simulink library "tqd"  (R2021b)
settings: Solver=VariableStepAuto  StartTime=0.0  StopTime=10.0  RelTol=1e-3
undefined symbols (not defined in the file or in its folder): ATQD_APSDecReq_X_kph, ATQD_APSDecReq_Y_mps2, ATQD_APSDecReqCMD_X_kph, ATQD_APSDecReqTs_X_pct, ATQD_APSDecTimeGain_X_Deg, ATQD_APSDecTimeGain_Y_s, ATQD_APSReqLowSpd_X_Deg, ATQD_AutoHoldReleaseBPS_X_Deg, ATQD_AWDLoadTrqnsGain_X_kg, ATQD_AWDLoadTrqnsGain_Y_pct, ATQD_BOSEnBPSPosn_X_kph, ATQD_BOSMap_X_rpm, ATQD_BOSMap_Y_pct, ATQD_CreepBaseTqD_X_kph, ATQD_CreepBaseTqD_Y_Deg, ATQD_CreepBaseTqR_X_kph, ATQD_CreepBaseTqR_Y_Deg, ATQD_CreepBPSDisPosn_X_Deg, ATQD_CreepBPSDisPosnR_X_Deg, ATQD_CreepBPSEnPosn_X_Deg, ATQD_CreepBPSEnPosnR_X_Deg, ATQD_CreepDeltaTq_X_kph, ATQD_CreepIterm_X_kph, ATQD_CreepIterm_Y_kph, ATQD_CreepItermMaxLimit_X_pct, ATQD_CreepPreloadTime_X_kph, ATQD_CreepPreloadTq_X_kph, ATQD_CreepPreloadTq_Y_s, ATQD_CreepProtTq_X_Deg, ATQD_CreepPterm_X_kph, ATQD_CreepPterm_Y_kph, ATQD_ECOTqMapD_X_rpm, ATQD_ECOTqMapD_Y_pct, ATQD_EOPDTqMapDCon_X_rpm, ATQD_EOPDTqMapDCon_Y_Deg, ATQD_EstInitVehWeight_X_c, ATQD_LHMRollGenMapD_X_rpm, ATQD_LHMRollGenMapD_Y_rpm, ATQD_LHMTqMapD_X_rpm, ATQD_LHMTqMapD_Y_pct, ATQD_NL1TqMapD_X_rpm, ATQD_NL1TqMapD_Y_pct, ATQD_NOPDTqMapDCon_X_rpm, ATQD_NOPDTqMapDCon_Y_Deg, ATQD_NRMRrEDUSpRat_X_rpm, ATQD_NRMRrEDUSpRat_Y_Nm, ATQD_OPDHoldDownRelDelay_X_Deg, ATQD_OPDHoldEnSpd_X_Deg, ATQD_OPDHoldRelDetTime_X_Deg, ATQD_OPDHoldReleaseTq_X_Deg, ATQD_OrigPedTqLowLim_X_Deg, ATQD_OrigPedTqLowLim_Y_pct, ATQD_PedalMapClimbUpLim_X_rpm, ATQD_PedalMapClimbUpLim_Y_Deg, ATQD_PreLoadTq_X_s, ATQD_RollGenMapEL1_X_rpm, ATQD_RollGenMapEL1_Y_rpm, ATQD_SL1TqMapD_X_rpm, ATQD_SL1TqMapD_Y_pct, ATQD_SlideRegenTqGain_X_Gps ... (+487)
libraries: hcu_lib x83, simulink x73, tqr x1
(part 10 of 19)

== system tqd/TQD/TorqueDemand/Signal_convert/VehWeightEst/Desicion ==
  task_time_s : Inport
  VTQD_VehWeightEstDis_flg : Inport  Port=2
  VTQD_EstVehWeight_kg : Inport  Port=3
  VINP_DriverSeatBeltCmd_flg : Inport  Port=4
  VINP_PsngrSeatBeltCmd_flg : Inport  Port=5
  VINP_RDriverSeatBeltCmd_flg : Inport  Port=6
  VINP_RCenterSeatBeltCmd_flg : Inport  Port=7
  VINP_RPsngrSeatBeltCmd_flg : Inport  Port=8
  VTQD_EstLongAccCheckPass_flg : Inport  Port=9
  VTQD_EstFrRealTqCheckPass_flg : Inport  Port=10
  VTQD_EstRrRealTqCheckPass_flg : Inport  Port=11
  AND : Logic  Inputs=5  AllPortsSameDT=off  OutDataTypeStr=boolean
  Add : Sum  Inputs=+++++
  Constant1 : Constant  Value=eps
  Constant{2,4,6,8,10} (5 alike) : Constant  Value=ZERO_INT
  Constant{3,5,7,9,11} (5 alike) : Constant  Value=ONE_INT
  Constant12 : Constant  Value=KTQD_EstEndDelayTime_s
  Data Type Conversion : DataTypeConversion  OutDataTypeStr=single
  Delay : Delay  DelayLength=1
  Delay1 : Delay  DelayLength=1
  DelayEnable : hcu_lib/Basic_Blocks/DelayEnable
  Equal : RelationalOperator  OutDataTypeStr=boolean  RndMeth=Simplest
  MTQD_EstInitVehWeight_Y_kg : Lookup_n-D  NumberOfTableDimensions=1  BreakpointsForDimension1=ATQD_EstInitVehWeight_X_c  Table=MTQD_EstInitVehWeight_Y_kg  ExtrapMethod=Clip  InternalRulePriority=Speed  RndMeth=Simplest  InputSameDT=on
  NOT : Logic  Operator=NOT  AllPortsSameDT=off  OutDataTypeStr=boolean
  Switch{,1..6} (7 alike) : Switch  Criteria=u2 > Threshold
  VTQD_VehWeightEstEnd_flg : Outport
  VTQD_EstVehWeightResult_kg : Outport  Port=2
  wires:
  Constant7/1 -> Switch4/1
  Constant1/1 -> Equal/2
  Switch2/1 -> Add/1
  [VINP_DriverSeatBeltCmd_flg] -> Switch2/2
  [VINP_RCenterSeatBeltCmd_flg] -> Switch4/2
  Switch5/1 -> Add/4
  Equal/1 -> Switch1/2
  Constant10/1 -> Switch6/3
  [VTQD_VehWeightEstDis_flg] -> AND/1
  Switch6/1 -> Add/5
  Delay/1 -> NOT/1
  Switch3/1 -> Add/2
  Constant6/1 -> Switch4/3
  Constant3/1 -> Switch2/1
  [VTQD_EstActVehWeight_kg] -> Switch1/1
  Constant2/1 -> Switch2/3
  [VTQD_VehWeightEstEnter_flg] -> Switch/2
  Constant11/1 -> Switch6/1
  Switch1/1 -> [VTQD_EstVehWeightResult_kg]  "VTQD_EstVehWeightResult_kg"
  Constant4/1 -> Switch3/3
  Constant5/1 -> Switch3/1
  [VINP_RDriverSeatBeltCmd_flg] -> Switch5/2
  Switch/1 -> Delay1/1, [VTQD_EstActVehWeight_kg]  "VTQD_EstActVehWeight_kg"
  AND/1 -> [VTQD_VehWeightEstEnter_flg]  "VTQD_VehWeightEstEnter_flg"
  [VINP_RPsngrSeatBeltCmd_flg] -> Switch6/2
  [VTQD_EstActVehWeight_kg] -> Equal/1
  [VINP_PsngrSeatBeltCmd_flg] -> Switch3/2
  Delay1/1 -> Switch/3
  [VTQD_EstInitVehWeight_kg] -> Switch1/3
  Constant9/1 -> Switch5/1
  Constant8/1 -> Switch5/3
  [VTQD_EstVehWeight_kg] -> Switch/1
  [VTQD_VehWeightEstEnd_flg] -> Delay/1
  NOT/1 -> AND/2
  Switch4/1 -> Add/3
  [VTQD_VehWeightEstDis_flg] -> DelayEnable/1
  Constant12/1 -> DelayEnable/2
  [task_time_s] -> DelayEnable/3
  DelayEnable/1 -> [VTQD_VehWeightEstEnd_flg]  "VTQD_VehWeightEstEnd_flg"
  task_time_s/1 -> [task_time_s]
  [VTQD_VehWeightEstEnd_flg] -> VTQD_VehWeightEstEnd_flg/1
  VTQD_VehWeightEstDis_flg/1 -> [VTQD_VehWeightEstDis_flg]
  VTQD_EstVehWeight_kg/1 -> [VTQD_EstVehWeight_kg]
  [VTQD_EstVehWeightResult_kg] -> VTQD_EstVehWeightResult_kg/1
  VINP_DriverSeatBeltCmd_flg/1 -> [VINP_DriverSeatBeltCmd_flg]
  VINP_PsngrSeatBeltCmd_flg/1 -> [VINP_PsngrSeatBeltCmd_flg]
  VINP_RDriverSeatBeltCmd_flg/1 -> [VINP_RDriverSeatBeltCmd_flg]
  VINP_RCenterSeatBeltCmd_flg/1 -> [VINP_RCenterSeatBeltCmd_flg]
  VINP_RPsngrSeatBeltCmd_flg/1 -> [VINP_RPsngrSeatBeltCmd_flg]
  VTQD_EstRrRealTqCheckPass_flg/1 -> [VTQD_EstRrRealTqCheckPass_flg]
  VTQD_EstFrRealTqCheckPass_flg/1 -> [VTQD_EstFrRealTqCheckPass_flg]
  VTQD_EstLongAccCheckPass_flg/1 -> [VTQD_EstLongAccCheckPass_flg]
  [VTQD_EstLongAccCheckPass_flg] -> AND/3
  [VTQD_EstFrRealTqCheckPass_flg] -> AND/4
  [VTQD_EstRrRealTqCheckPass_flg] -> AND/5
  MTQD_EstInitVehWeight_Y_kg/1 -> [VTQD_EstInitVehWeight_kg]  "VTQD_EstInitVehWeight_kg"
  Data Type Conversion/1 -> MTQD_EstInitVehWeight_Y_kg/1
  Add/1 -> Data Type Conversion/1  "VTQD_EstInitVehWightX_c"

== system tqd/TQD/TorqueDemand/TorqueModule/AvaliableTqLimit/If Action Subsystem1 ==
  VTQD_WhlTqCapGenF_Nm : Inport
  VTQD_WhlTqCapGenR_Nm : Inport  Port=2
  VTQD_DriverWhlTqDemFr_Nm : Inport  Port=3
  VTQD_DriverWhlTqDemRr_Nm : Inport  Port=4
  VVMC_ADASActive_flg : Inport  Port=5
  Action Port : ActionPort
  Constant{,1..3} (4 alike) : Constant  Value=ZERO_FLOAT
  Data Type Conversion1 : DataTypeConversion  OutDataTypeStr=single
  Data Type Conversion5 : DataTypeConversion  OutDataTypeStr=single
  Display : Display
  Display1 : Display
  Subtract : Sum  Inputs=+-
  Subtract1 : Sum  Inputs=+-
  Switch : Switch  Criteria=u2 > Threshold
  Switch1 : Switch  Criteria=u2 > Threshold
  Switch2 : Switch  Criteria=u2 ~= 0
  Switch3 : Switch  Criteria=u2 ~= 0
  VTQD_AvailTqWithARgnFr_Nm : Outport
  VTQD_AvailTqWithARgnRr_Nm : Outport  Port=2
  wires:
  Constant1/1 -> Switch1/1
  Constant/1 -> Switch/1
  Subtract1/1 -> Switch1/2, Switch1/3
  Subtract/1 -> Switch/2, Switch/3
  Switch1/1 -> Data Type Conversion5/1, VTQD_AvailTqWithARgnRr_Nm/1
  Switch/1 -> Data Type Conversion1/1, VTQD_AvailTqWithARgnFr_Nm/1
  VTQD_WhlTqCapGenR_Nm/1 -> Subtract1/1
  VTQD_WhlTqCapGenF_Nm/1 -> Subtract/1
  VTQD_DriverWhlTqDemFr_Nm/1 -> Switch2/3
  Switch2/1 -> Subtract/2
  Constant2/1 -> Switch2/1
  VVMC_ADASActive_flg/1 -> Switch3/2, Switch2/2
  Constant3/1 -> Switch3/1
  VTQD_DriverWhlTqDemRr_Nm/1 -> Switch3/3
  Switch3/1 -> Subtract1/2
  Data Type Conversion1/1 -> Display/1  "VTQD_AvailTqWithARgnFr_Nm"
  Data Type Conversion5/1 -> Display1/1  "VTQD_AvailTqWithARgnRr_Nm"

== system tqd/TQD/TorqueDemand/TorqueModule/AvaliableTqLimit/If Action Subsystem2 ==
  VTQD_WhlTqCapGenF_Nm : Inport
  VTQD_WhlTqCapGenR_Nm : Inport  Port=2
  Action Port : ActionPort
  Data Type Conversion4 : DataTypeConversion  OutDataTypeStr=single
  Data Type Conversion5 : DataTypeConversion  OutDataTypeStr=single
  Display : Display
  Display1 : Display
  VTQD_AvailTqNoARgnFr_Nm : Outport
  VTQD_AvailTqNoARgnRr_Nm : Outport  Port=2
  wires:
  VTQD_WhlTqCapGenF_Nm/1 -> Data Type Conversion4/1, VTQD_AvailTqNoARgnFr_Nm/1
  VTQD_WhlTqCapGenR_Nm/1 -> Data Type Conversion5/1, VTQD_AvailTqNoARgnRr_Nm/1
  Data Type Conversion4/1 -> Display/1  "VTQD_AvailTqNoARgnFr_Nm"
  Data Type Conversion5/1 -> Display1/1  "VTQD_AvailTqNoARgnRr_Nm"

== system tqd/TQD/TorqueDemand/TorqueModule/AvaliableTqLimit/TorqueCapacityCalcalation ==
  VTQD_FrShaftSpd_rpm : Inport
  VTQD_RrShaftSpd_rpm : Inport  Port=2
  VINP_HVBPwrAvailDchrg_kw : Inport  Port=3
  VINP_HVBPwrAvailChrg_kw : Inport  Port=4
  KTQD_FrBatapCont_factor : Inport  Port=5
  KTQD_RrBatapCont_factor : Inport  Port=6
  VTQD_FrEDUSpRat_cmd : Inport  Port=7
  VTQD_RrEDUSpRat_rat : Inport  Port=8
  VINP_FrMotorAvailTq_Nm : Inport  Port=9
  VINP_RrMotorAvailTq_Nm : Inport  Port=10
  VINP_HVBCellVoltMax_mV : Inport  Port=11
  VINP_HVBCellVoltMin_mV : Inport  Port=12
  VINP_HVBSOH_pct : Inport  Port=13
  VINP_FrRegenAvailTq_Nm : Inport  Port=14
  VINP_RrRegenAvailTq_Nm : Inport  Port=15
  VTQD_GearActualPosn_enum : Inport  Port=16
  VINP_VehicleType_enum : Inport  Port=17
  CapacityDistribution : Subsystem
  Generation : Subsystem
  Motoring : Subsystem
  TMAvailablePwr_Calculation : Subsystem
  VTQD_WhlTqCapMotFr_Nm : Outport
  VTQD_WhlTqCapMotRr_Nm : Outport  Port=2
  VTQD_WhlTqCapGenFr_Nm : Outport  Port=3
  VTQD_WhlTqCapGenRr_Nm : Outport  Port=4
  wires:
  [VTQD_TMPwrAvailDchrg_kW] -> CapacityDistribution/3(VTQD_TMPwrAvailDchrg_kW)
  TMAvailablePwr_Calculation/1(VTQD_TMPwrAvailDchrg_kW) -> [VTQD_TMPwrAvailDchrg_kW]
  [VINP_HVBPwrAvailDchrg_kw] -> TMAvailablePwr_Calculation/1(VINP_HVBPwrAvailDchrg_kw)
  Motoring/2(VTQD_WhlTqCapMotRr_Nm) -> VTQD_WhlTqCapMotRr_Nm/1
  [VTQD_RrEDUSpRat_rat] -> CapacityDistribution/2(VTQD_RrEDUSpRat_rat)
  [VTQD_FrEDUSpRat_rat] -> CapacityDistribution/1(VTQD_FrEDUSpRat_cmd)
  CapacityDistribution/4(VTQD_RrHVBPwrAvailChrg_kw) -> [VTQD_RrHVBPwrAvailChrg_kw]
  CapacityDistribution/3(VTQD_FrHVBPwrAvailChrg_kw) -> [VTQD_FrHVBPwrAvailChrg_kw]
  CapacityDistribution/2(VTQD_RrHVBPwrAvailDchrg_kw) -> [VTQD_RrHVBPwrAvailDchrg_kw]
  CapacityDistribution/1(VTQD_FrHVBPwrAvailDchrg_kw) -> [VTQD_FrHVBPwrAvailDchrg_kw]
  [VINP_HVBPwrAvailChrg_kw] -> CapacityDistribution/4(VINP_HVBPwrAvailChrg_kw)
  [VTQD_RrHVBPwrAvailChrg_kw] -> Generation/4(VTQD_RrHVBPwrAvailChrg_kw)
  [KTQD_RrBatapCont_factor] -> Generation/6(KTQD_RrBatapCont_factor)
  [VTQD_FrShaftSpd_rpm] -> Generation/1(VTQD_FrShaftSpd_rpm)
  [VTQD_FrHVBPwrAvailChrg_kw] -> Generation/3(VTQD_FrHVBPwrAvailChrg_kw)
  [VTQD_RrShaftSpd_rpm] -> Generation/2(VTQD_RrShaftSpd_rpm)
  [KTQD_FrBatapCont_factor] -> Generation/5(KTQD_FrBatapCont_factor)
  Generation/1(VTQD_WhlTqCapGenFr_Nm) -> VTQD_WhlTqCapGenFr_Nm/1
  Generation/2(VTQD_WhlTqCapGenRr_Nm) -> VTQD_WhlTqCapGenRr_Nm/1
  [VTQD_RrHVBPwrAvailDchrg_kw] -> Motoring/4(VTQD_RrHVBPwrAvailDchrg_kw)
  [VTQD_FrHVBPwrAvailDchrg_kw] -> Motoring/3(VTQD_FrHVBPwrAvailDchrg_kw)
  [KTQD_RrBatapCont_factor] -> Motoring/6(KTQD_RrBatapCont_factor)
  VTQD_RrEDUSpRat_rat/1 -> [VTQD_RrEDUSpRat_rat]
  VTQD_FrEDUSpRat_cmd/1 -> [VTQD_FrEDUSpRat_rat]
  KTQD_RrBatapCont_factor/1 -> [KTQD_RrBatapCont_factor]
  [VTQD_RrShaftSpd_rpm] -> Motoring/2(VTQD_RrShaftSpd_rpm)
  VTQD_RrShaftSpd_rpm/1 -> [VTQD_RrShaftSpd_rpm]
  VTQD_FrShaftSpd_rpm/1 -> [VTQD_FrShaftSpd_rpm]
  VINP_HVBPwrAvailChrg_kw/1 -> [VINP_HVBPwrAvailChrg_kw]
  VINP_HVBPwrAvailDchrg_kw/1 -> [VINP_HVBPwrAvailDchrg_kw]
  KTQD_FrBatapCont_factor/1 -> [KTQD_FrBatapCont_factor]
  [VTQD_FrShaftSpd_rpm] -> Motoring/1(VTQD_FrShaftSpd_rpm)
  Motoring/1(VTQD_WhlTqCapMotFr_Nm) -> VTQD_WhlTqCapMotFr_Nm/1
  [KTQD_FrBatapCont_factor] -> Motoring/5(KTQD_FrBatapCont_factor)
  VINP_HVBSOH_pct/1 -> [VINP_HVBSOH_pct]
  VINP_HVBCellVoltMin_mV/1 -> [VINP_HVBCellVoltMin_mV]
  VINP_HVBCellVoltMax_mV/1 -> [VINP_HVBCellVoltMax_mV]
  [VINP_HVBSOH_pct] -> Motoring/9(VINP_HVBSOH_pct)
  [VINP_HVBCellVoltMin_mV] -> Motoring/8(VINP_HVBCellVoltMin_mV)
  [VINP_HVBCellVoltMax_mV] -> Motoring/7(VINP_HVBCellVoltMax_mV)
  [VINP_RrMotorAvailTq_Nm] -> Motoring/11(VINP_RrMotorAvailTq_Nm)
  [VINP_FrMotorAvailTq_Nm] -> Motoring/10(VINP_FrMotorAvailTq_Nm)
  [VINP_FrRegenAvailTq_Nm] -> Generation/7(VINP_FrRegenAvailTq_Nm)
  [VINP_RrRegenAvailTq_Nm] -> Generation/8(VINP_RrRegenAvailTq_Nm)
  VINP_RrRegenAvailTq_Nm/1 -> [VINP_RrRegenAvailTq_Nm]
  VINP_FrRegenAvailTq_Nm/1 -> [VINP_FrRegenAvailTq_Nm]
  VINP_FrMotorAvailTq_Nm/1 -> [VINP_FrMotorAvailTq_Nm]
  VINP_RrMotorAvailTq_Nm/1 -> [VINP_RrMotorAvailTq_Nm]
  [VTQD_GearActualPosn_enum] -> Motoring/12(VTQD_GearActualPosn_enum)
  [VTQD_GearActualPosn_enum] -> Generation/9(VTQD_GearActualPosn_enum)
  VTQD_GearActualPosn_enum/1 -> [VTQD_GearActualPosn_enum]
  [VINP_VehicleType_enum] -> Motoring/13(VINP_VehicleType_enum)
  [VINP_VehicleType_enum] -> Generation/10(VINP_VehicleType_enum)
  VINP_VehicleType_enum/1 -> [VINP_VehicleType_enum]

== system tqd/TQD/TorqueDemand/TorqueModule/DriverWhlTqDem/BOS ==
  VTQD_ActBPSPosn_pct : Inport
  VTQD_TqTargetShaftSpd_rpm : Inport  Port=2
  VTQD_VehActSpd_kph : Inport  Port=3
  VTQD_PedalMapWhlTq_Nm : Inport  Port=4
  VTQD_CreepBaseTqR_Nm : Inport  Port=5
  VTQD_CreepBaseTqD_Nm : Inport  Port=6
  VTQD_GearActualPosn_enum : Inport  Port=7
  VVMC_APSActive_flg : Inport  Port=8
  VTQD_LowIdleAccPedal_flg : Inport  Port=9
  VTQD_HighBPSPosn_flg : Inport  Port=10
  VTQD_BrkSwSta_flg : Inport  Port=11
  AND : Logic  Inputs=4  AllPortsSameDT=off  OutDataTypeStr=boolean
  AND1 : Logic  AllPortsSameDT=off  OutDataTypeStr=boolean
  AND2 : Logic  AllPortsSameDT=off  OutDataTypeStr=boolean
  Constant1 : Constant  Value=KTQD_BOSEnPedalTq_Nm
  Constant18 : Constant  Value=ZERO_FLOAT
  Constant20 : Constant  Value=ENUM_GEARACTUALPOSN_R
  Constant3 : Constant  Value=ONE_PERCENT
  Detect Change : simulink/Logic and Bit Operations/Detect Change  vinit=0  OutDataTypeStr=boolean
  Equal10 : RelationalOperator  Operator===  OutDataTypeStr=boolean  RndMeth=Simplest
  MTQD_BOSEnBPSPosn_Y_pct : Lookup_n-D  NumberOfTableDimensions=1  BreakpointsForDimension1=ATQD_BOSEnBPSPosn_X_kph  Table=MTQD_BOSEnBPSPosn_Y_pct  InternalRulePriority=Speed  RndMeth=Simplest  InputSameDT=on
  MTQD_BOSMap_Z_pct : Lookup_n-D  BreakpointsForDimension1=ATQD_BOSMap_Y_pct  BreakpointsForDimension2=ATQD_BOSMap_X_rpm  Table=MTQD_BOSMap_Z_pct  ExtrapMethod=Clip  InternalRulePriority=Speed  RndMeth=Simplest  InputSameDT=on
      settings: InputPortMap=u0,u1
  Max : MinMax  Function=max  Inputs=2
  NOT{,1..3} (4 alike) : Logic  Operator=NOT  AllPortsSameDT=off  OutDataTypeStr=boolean
  OR : Logic  Operator=OR  Inputs=3  AllPortsSameDT=off  OutDataTypeStr=boolean
  OR1 : Logic  Operator=OR  AllPortsSameDT=off  OutDataTypeStr=boolean
  Product1 : Product  RndMeth=Zero
  Product2 : Product  RndMeth=Zero
  Product3 : Product  RndMeth=Zero
  Relational Operator : RelationalOperator  Operator=>  OutDataTypeStr=boolean  RndMeth=Simplest
  Relational Operator1 : RelationalOperator  Operator=>  OutDataTypeStr=boolean  RndMeth=Simplest
  Relational Operator2 : RelationalOperator  OutDataTypeStr=boolean  RndMeth=Simplest
  Relational Operator5 : RelationalOperator  Operator=>  OutDataTypeStr=boolean  RndMeth=Simplest
  SR_Latch : hcu_lib/Basic_Blocks/SR_Latch
  Switch7 : Switch  Criteria=u2 > Threshold
  Switch8 : Switch  Criteria=u2 > Threshold
  VTQD_BOSEnable_flg : Outport
  VTQD_BOSTq_Nm : Outport  Port=2
  wires:
  VTQD_TqTargetShaftSpd_rpm/1 -> [VTQD_TqTargetShaftSpd_rpm]
  [VTQD_ActBPSPosn_pct] -> MTQD_BOSMap_Z_pct/1
  [VTQD_TqTargetShaftSpd_rpm] -> MTQD_BOSMap_Z_pct/2
  Constant3/1 -> Product1/2
  Product1/1 -> [VTQD_BOSReduction_gain]  "VTQD_BOSReduction_gain"
  MTQD_BOSMap_Z_pct/1 -> Product1/1
  VTQD_ActBPSPosn_pct/1 -> [VTQD_ActBPSPosn_pct]
  Relational Operator/1 -> AND/1
  VTQD_VehActSpd_kph/1 -> [VTQD_VehActSpd_kph]
  [VTQD_VehActSpd_kph] -> MTQD_BOSEnBPSPosn_Y_pct/1
  MTQD_BOSEnBPSPosn_Y_pct/1 -> Relational Operator/2  "VTQD_BOSEnBPSPosn_pct"
  [VTQD_ActBPSPosn_pct] -> Relational Operator/1
  VTQD_PedalMapWhlTq_Nm/1 -> [VTQD_PedalMapWhlTq_Nm]
  Relational Operator1/1 -> AND/2
  [VTQD_PedalMapWhlTq_Nm] -> Relational Operator1/1
  Constant1/1 -> Relational Operator1/2
  [VTQD_PedalMapWhlTq_Nm] -> Product2/1
  [VTQD_BOSReduction_gain] -> Product2/2
  Product3/1 -> Max/2
  Switch8/1 -> VTQD_BOSTq_Nm/1, [VTQD_BOSTq_Nm]  "VTQD_BOSTq_Nm"
  [VTQD_CreepBaseTqR_Nm] -> Switch7/1
  Max/1 -> Switch8/1
  Product2/1 -> Switch8/3
  Equal10/1 -> Switch7/2
  [VTQD_PedalMapWhlTq_Nm] -> Product3/1
  [VTQD_BOSReduction_gain] -> Product3/2
  [VTQD_GearActualPosn_enum] -> Equal10/1
  Relational Operator5/1 -> Switch8/2
  Constant20/1 -> Equal10/2
  Switch7/1 -> Max/1
  Constant18/1 -> Relational Operator5/2
  [VTQD_CreepBaseTqD_Nm] -> Switch7/3
  VTQD_CreepBaseTqD_Nm/1 -> [VTQD_CreepBaseTqD_Nm]
  VTQD_CreepBaseTqR_Nm/1 -> [VTQD_CreepBaseTqR_Nm]
  VTQD_GearActualPosn_enum/1 -> [VTQD_GearActualPosn_enum]
  [VTQD_BOSReduction_gain] -> Relational Operator5/1
  NOT/1 -> AND/3
  [VVMC_APSActive_flg] -> NOT/1
  VVMC_APSActive_flg/1 -> [VVMC_APSActive_flg]
  VTQD_LowIdleAccPedal_flg/1 -> [VTQD_LowIdleAccPedal_flg]
  [VTQD_LowIdleAccPedal_flg] -> NOT2/1
  NOT2/1 -> AND/4
  [VTQD_BrkSwSta_flg] -> NOT3/1
  AND2/1 -> OR/3
  AND1/1 -> OR1/1
  Detect Change/1 -> OR1/2
  Relational Operator2/1 -> OR/1
  [VTQD_LowIdleAccPedal_flg] -> AND2/1
  [VTQD_GearActualPosn_enum] -> Detect Change/1
  OR1/1 -> SR_Latch/2
  NOT3/1 -> AND2/2
  SR_Latch/1 -> VTQD_BOSEnable_flg/1  "VTQD_BOSEnable_flg"
  AND/1 -> NOT1/1, SR_Latch/1
  [VTQD_HighBPSPosn_flg] -> OR/2
  OR/1 -> AND1/2
  NOT1/1 -> AND1/1
  [VTQD_PedalMapWhlTq_Nm] -> Relational Operator2/1
  [VTQD_BOSTq_Nm] -> Relational Operator2/2
  VTQD_BrkSwSta_flg/1 -> [VTQD_BrkSwSta_flg]
  VTQD_HighBPSPosn_flg/1 -> [VTQD_HighBPSPosn_flg]

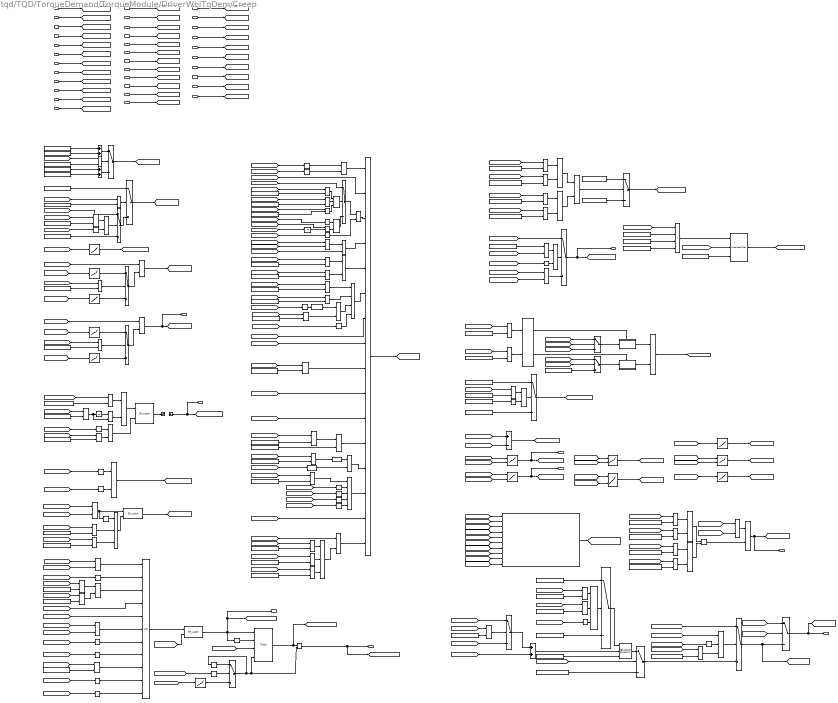
== system tqd/TQD/TorqueDemand/TorqueModule/DriverWhlTqDem/Creep ==
  note: Creep Enable Judgement
  note: Vehicle Actual Speed Calculation
  note: Creep Wheel Torque Demand Calculation
  VTQD_CreepON_flg : Inport
  VTQD_GearActualPosn_enum : Inport  Port=2
  VTQD_LowIdleAccPedal_flg : Inport  Port=3
  VINP_VehSpeed_kph : Inport  Port=4
  VTQD_TMRotateDirction_enum : Inport  Port=5
  VTQD_RegenMode_enum : Inport  Port=6
  VTQD_ActBPSPosn_pct : Inport  Port=7
  VTQD_PedalMapWhlTq_Nm : Inport  Port=8
  VINP_RrRBCActive_flg : Inport  Port=9
  VINP_FrRBCActive_flg : Inport  Port=10
  VVMC_ADASActive_flg : Inport  Port=11
  task_time_s : Inport  Port=12
  VTQD_LoSpdBrkCtrl_flg : Inport  Port=13
  VINP_AVHActive_flg : Inport  Port=14
  VTQD_APSReq_enum : Inport  Port=15
  VVMC_APSSpeedCMD_kph : Inport  Port=16
  VVMC_APSActive_flg : Inport  Port=17
  VTQD_RDCActive_enum : Inport  Port=18
  VVMC_APSReq_enum : Inport  Port=19
  " VINP_FrEDURealTMTq_Nm" : Inport  Port=20
  VINP_RrEDURealTMTq_Nm : Inport  Port=21
  VTQD_PreLoadPreEn_flg : Inport  Port=22
  VVMC_EstSlope_Deg : Inport  Port=23
  VPMM_PwrSta_enum : Inport  Port=24
  VTQD_TqTargetShaftSpd_rpm : Inport  Port=25
  VTQD_APSReqTimer_s : Inport  Port=26
  VINP_EPBSta_enum : Inport  Port=27
  VTQD_OPDHoldEnRel_flg : Inport  Port=28
  VTQD_ActAPSPosn_pct : Inport  Port=29
  VVMC_CAASActive_flg : Inport  Port=30
  VDDM_EPB1NoComCFS_flg : Inport  Port=31
  VDDM_EPB1RCErrCFS_flg : Inport  Port=32
  VDDM_EPB1CSErrCFS_flg : Inport  Port=33
  VDDM_EPBSigErrCFS_flg : Inport  Port=34
  AND{,1..2,4..7,9,11..12,15..16} (12 alike) : Logic  AllPortsSameDT=off  OutDataTypeStr=boolean
  AND10 : Logic  Operator=OR  AllPortsSameDT=off  OutDataTypeStr=boolean
  AND{3,8,13..14} (4 alike) : Logic  Inputs=3  AllPortsSameDT=off  OutDataTypeStr=boolean
  Add : Sum  Inputs=+-
  Add1 : Sum
  Add2 : Sum
  Add4 : Sum
  Constant1 : Constant  Value=KTQD_APSCMDEnCreepSpd_kph
  Constant10 : Constant  Value=KTQD_CreepTargetSpdR_kph
  Constant{3,11..12,21,25,58,62} (7 alike) : Constant  Value=ENUM_GEARACTUALPOSN_D
  Constant13 : Constant  Value=KTQD_CreepEnableSpd_kph
  Constant14 : Constant  Value=RPM2RADPS
  Constant15 : Constant  Value=ZERO_FLOAT
  Constant16 : Constant  Value=KTQD_TireRadius_m
  Constant17 : Constant  Value=ENUM_RDCACTSTA_NOREQUEST
  Constant18 : Constant  Value=ENUM_APSREQ_DECELCTRL  OutDataTypeStr=uint8
  Constant19 : Constant  Value=MPS2KPH
  Constant{2,9,20,31,35..36,38,42..44} (10 alike) : Constant  Value=ENUM_GEARACTUALPOSN_R
  Constant22 : Constant  Value=KTQD_CreepLowLimitTq_Nm
  Constant23 : Constant  Value=KTQD_CreepPrLoadEnSpd_kph
  Constant24 : Constant  Value=ENUM_RDCACTSTA_NOREQUEST
  Constant26 : Constant  Value=KTQD_CreepDisableSpdofst_kph
  Constant27 : Constant  Value=KTQD_CreepEnableSpdR_kph
  Constant28 : Constant  Value=KTQD_CreepDisableSpdofstR_kph
  Constant29 : Constant  Value=KTQD_CreepEnableSpdR_kph
  Constant30 : Constant  Value=ENUM_TMROTATEDIRECTACT_REVERSE  OutDataTypeStr=Inherit: Inherit via back propagation
  Constant32 : Constant  Value=ENUM_TMROTATEDIRECTACT_FORWARD  OutDataTypeStr=Inherit: Inherit via back propagation
  Constant33 : Constant  Value=KTQD_VehActSpdNegGain_gain
  Constant34 : Constant  Value=KTQD_VehActSpdPosGain_gain
  Constant37 : Constant  Value=ENUM_TMROTATEDIRECTACT_REVERSE  OutDataTypeStr=Inherit: Inherit via back propagation
  Constant39 : Constant  Value=ENUM_TMROTATEDIRECTACT_FORWARD  OutDataTypeStr=Inherit: Inherit via back propagation
  Constant{4,8,52,54,59,64} (6 alike) : Constant  Value=ENUM_REGENLEVEL_OPD
  Constant40 : Constant  Value=KTQD_RBCCreepRecTq_Nm
  Constant41 : Constant  Value=KTQD_RBCCreepRecTq_Nm
  Constant45 : Constant  Value=ENUM_POWERSTA_READY
  Constant46 : Constant  Value=KTQD_CreepEnableSpd_kph
  Constant47 : Constant  Value=KTQD_RPM2VehSpdTs_c
  Constant48 : Constant  Value=KTQD_CreepVehSpdSW_flg
  Constant49 : Constant  Value=KTQD_CreepTargetSpdD_kph
  Constant5 : Constant  Value=ENUM_APSREQ_BRKHOLD  OutDataTypeStr=uint8
  Constant50 : Constant  Value=KTQD_OPDCreepTargetSpdD_kph
  Constant51 : Constant  Value=KTQD_APSReqDisCreep_flg  OutDataTypeStr=uint8
  Constant53 : Constant  Value=KTQD_APSReqDelayTime_s
  Constant55 : Constant  Value=ENUM_EPBSTA_APPLIED  OutDataTypeStr=uint8
  Constant56 : Constant  Value=KTQD_APSReqDisCreep_flg
  Constant57 : Constant  Value=KTQD_CreepUpLimitTq_Nm
  Constant6 : Constant  Value=ENUM_GEARACTUALPOSN_P
  Constant60 : Constant  Value=KTQD_OPDCreepDUpLimitTq_Nm
  Constant61 : Constant  Value=KTQD_CreepDisPedTqSpd_kph
  Constant63 : Constant  Value=KTQD_CreepAPSPosn2Launch_pct
  Constant65 : Constant  Value=ENUM_APSREQ_DECELCTRL  OutDataTypeStr=uint8
  Constant7 : Constant  Value=ENUM_GEARACTUALPOSN_N
  Data Type Conversion : DataTypeConversion
  Delay : Delay  DelayLength=1
  Delay1 : Delay  DelayLength=1
  Detect Change : simulink/Logic and Bit Operations/Detect Change  vinit=0  OutDataTypeStr=boolean
  Detect Increase : simulink/Logic and Bit Operations/Detect Increase  vinit=0.0  OutDataTypeStr=boolean
  Equal{,1..4,6..8,10..16,19..31,33..39} (35 alike) : RelationalOperator  Operator===  OutDataTypeStr=boolean  RndMeth=Simplest
  Equal17 : RelationalOperator  Operator=<=  OutDataTypeStr=boolean  RndMeth=Simplest
  Equal18 : RelationalOperator  Operator=~=  OutDataTypeStr=boolean  RndMeth=Simplest
  Equal32 : RelationalOperator  OutDataTypeStr=boolean  RndMeth=Simplest
  Equal5 : RelationalOperator  Operator=<=  OutDataTypeStr=boolean  RndMeth=Simplest
  Equal9 : RelationalOperator  Operator=<=  OutDataTypeStr=boolean  RndMeth=Simplest
  FirstOrderFilter : hcu_lib/Basic_Blocks/FirstOrderFilter
  GreaterThan : RelationalOperator  Operator=>  OutDataTypeStr=boolean  RndMeth=Simplest
  GreaterThan1 : RelationalOperator  Operator=>  OutDataTypeStr=boolean  RndMeth=Simplest
  GreaterThan2 : RelationalOperator  OutDataTypeStr=boolean  RndMeth=Simplest
  GreaterThan3 : RelationalOperator  Operator=>  OutDataTypeStr=boolean  RndMeth=Simplest
  GreaterThan4 : RelationalOperator  Operator=<=  OutDataTypeStr=boolean  RndMeth=Simplest
  Ground2 : Ground
  If : If  NumInputs=2  IfExpression=u1 ~= 0  ElseIfExpressions=u2 ~= 0  ShowElse=off
  If Action Subsystem : Subsystem  TreatAsAtomicUnit=on
  If Action Subsystem1 : Subsystem  TreatAsAtomicUnit=on
  LiuzgSwitch1 : Switch  Criteria=u2 ~= 0
      settings: AttributesFormatString=<%<Criteria>>
  Logical Operator{,2,4,6} (4 alike) : Logic  AllPortsSameDT=off  OutDataTypeStr=boolean
  Logical Operator1 : Logic  Operator=OR  AllPortsSameDT=off  OutDataTypeStr=boolean
  Logical Operator{8..11} (4 alike) : Logic  Operator=NOT  AllPortsSameDT=off  OutDataTypeStr=boolean
  Logical Operator3 : Logic  Inputs=11  AllPortsSameDT=off  OutDataTypeStr=boolean
  Logical Operator5 : Logic  Operator=OR  AllPortsSameDT=off  OutDataTypeStr=boolean
  Logical Operator7 : Logic  Inputs=5  AllPortsSameDT=off  OutDataTypeStr=boolean
  MTQD_CreepBPSDisPosnR_Y_pct : Lookup_n-D  NumberOfTableDimensions=1  BreakpointsForDimension1=ATQD_CreepBPSDisPosnR_X_Deg  Table=MTQD_CreepBPSDisPosnR_Y_pct  ExtrapMethod=Clip  InternalRulePriority=Speed  RndMeth=Simplest  InputSameDT=on
  MTQD_CreepBPSDisPosn_Y_pct : Lookup_n-D  NumberOfTableDimensions=1  BreakpointsForDimension1=ATQD_CreepBPSDisPosn_X_Deg  Table=MTQD_CreepBPSDisPosn_Y_pct  ExtrapMethod=Clip  InternalRulePriority=Speed  RndMeth=Simplest  InputSameDT=on
  MTQD_CreepBPSEnPosnR_Y_pct : Lookup_n-D  NumberOfTableDimensions=1  BreakpointsForDimension1=ATQD_CreepBPSEnPosnR_X_Deg  Table=MTQD_CreepBPSEnPosnR_Y_pct  ExtrapMethod=Clip  InternalRulePriority=Speed  RndMeth=Simplest  InputSameDT=on
  MTQD_CreepBPSEnPosn_Y_pct : Lookup_n-D  NumberOfTableDimensions=1  BreakpointsForDimension1=ATQD_CreepBPSEnPosn_X_Deg  Table=MTQD_CreepBPSEnPosn_Y_pct  ExtrapMethod=Clip  InternalRulePriority=Speed  RndMeth=Simplest  InputSameDT=on
  MTQD_CreepBaseTqD_Z_Nm : Lookup_n-D  BreakpointsForDimension1=ATQD_CreepBaseTqD_Y_Deg  BreakpointsForDimension2=ATQD_CreepBaseTqD_X_kph  Table=MTQD_CreepBaseTqD_Z_Nm  ExtrapMethod=Clip  InternalRulePriority=Speed  RndMeth=Simplest  InputSameDT=on
      settings: InputPortMap=u0,u1
  MTQD_CreepBaseTqR_Z_Nm : Lookup_n-D  BreakpointsForDimension1=ATQD_CreepBaseTqR_Y_Deg  BreakpointsForDimension2=ATQD_CreepBaseTqR_X_kph  Table=MTQD_CreepBaseTqR_Z_Nm  ExtrapMethod=Clip  InternalRulePriority=Speed  RndMeth=Simplest  InputSameDT=on
      settings: InputPortMap=u0,u1
  MTQD_CreepDeltaTq_Y_Nm : Lookup_n-D  NumberOfTableDimensions=1  BreakpointsForDimension1=ATQD_CreepDeltaTq_X_kph  Table=MTQD_CreepDeltaTq_Y_Nm  ExtrapMethod=Clip  InternalRulePriority=Speed  RndMeth=Simplest  InputSameDT=on
  MTQD_CreepIterm_Z_Nm : Lookup_n-D  BreakpointsForDimension1=ATQD_CreepIterm_Y_kph  BreakpointsForDimension2=ATQD_CreepIterm_X_kph  Table=MTQD_CreepIterm_Z_Nm  ExtrapMethod=Clip  InternalRulePriority=Speed  RndMeth=Simplest  InputSameDT=on
      settings: InputPortMap=u0,u1
  MTQD_CreepPrelaodTq_Z_Nm : Lookup_n-D  BreakpointsForDimension1=ATQD_CreepPreloadTq_Y_s  BreakpointsForDimension2=ATQD_CreepPreloadTq_X_kph  Table=MTQD_CreepPreloadTq_Z_Nm  ExtrapMethod=Clip  InternalRulePriority=Speed  RndMeth=Simplest  InputSameDT=on
      settings: InputPortMap=u0,u1
  MTQD_CreepPreloadTime_Y_s : Lookup_n-D  NumberOfTableDimensions=1  BreakpointsForDimension1=ATQD_CreepPreloadTime_X_kph  Table=MTQD_CreepPreloadTime_Y_s  ExtrapMethod=Clip  InternalRulePriority=Speed  RndMeth=Simplest  InputSameDT=on
  MTQD_CreepProtTq_Y_Nm : Lookup_n-D  NumberOfTableDimensions=1  BreakpointsForDimension1=ATQD_CreepProtTq_X_Deg  Table=MTQD_CreepProtTq_Y_Nm  ExtrapMethod=Clip  InternalRulePriority=Speed  RndMeth=Simplest  InputSameDT=on
  MTQD_CreepPterm_Z_Nm : Lookup_n-D  BreakpointsForDimension1=ATQD_CreepPterm_Y_kph  BreakpointsForDimension2=ATQD_CreepPterm_X_kph  Table=MTQD_CreepPterm_Z_Nm  ExtrapMethod=Clip  InternalRulePriority=Speed  RndMeth=Simplest  InputSameDT=on
      settings: InputPortMap=u0,u1
  MTQD_OPDHoldEnSpd_Y_kph : Lookup_n-D  NumberOfTableDimensions=1  BreakpointsForDimension1=ATQD_OPDHoldEnSpd_X_Deg  Table=MTQD_OPDHoldEnSpd_Y_kph  InternalRulePriority=Speed  RndMeth=Simplest  InputSameDT=on
  Merge : Merge
  NOT{,1..18} (19 alike) : Logic  Operator=NOT  AllPortsSameDT=off  OutDataTypeStr=boolean
  OR{,2..3,6..9} (7 alike) : Logic  Operator=OR  AllPortsSameDT=off  OutDataTypeStr=boolean
  OR1 : Logic  Operator=OR  Inputs=16  AllPortsSameDT=off  OutDataTypeStr=boolean
  OR4 : Logic  Inputs=4  AllPortsSameDT=off  OutDataTypeStr=boolean
  OR5 : Logic  Operator=OR  Inputs=3  AllPortsSameDT=off  OutDataTypeStr=boolean
  Product : Product
  Product1 : Product  Inputs=4
  Relational Operator : RelationalOperator  OutDataTypeStr=boolean  RndMeth=Simplest
  Relational Operator1 : RelationalOperator  Operator=<  OutDataTypeStr=boolean  RndMeth=Simplest
  Relational Operator2 : RelationalOperator  Operator=>  OutDataTypeStr=boolean  RndMeth=Simplest
  Relational Operator3 : RelationalOperator  Operator=>  OutDataTypeStr=boolean  RndMeth=Simplest
  Relational Operator4 : RelationalOperator  Operator=>  OutDataTypeStr=boolean  RndMeth=Simplest
  Relational Operator5 : RelationalOperator  Operator=<=  OutDataTypeStr=boolean  RndMeth=Simplest
  Relay : Relay  OnSwitchValue=KTQD_OPDCreepEnGrade_Deg  OffSwitchValue=KTQD_OPDCreepDisGrade_Deg  OnOutputValue=0  OffOutputValue=1
  Relay1 : Relay  OnSwitchValue=KTQD_CreepDisVehSpd_kph  OffSwitchValue=KTQD_CreepEnVehSpd_kph  OnOutputValue=0  OffOutputValue=1  OutDataTypeStr=boolean
  SR_Latch : hcu_lib/Basic_Blocks/SR_Latch
  SR_Latch1 : hcu_lib/Basic_Blocks/SR_Latch
  SR_Latch3 : hcu_lib/Basic_Blocks/SR_Latch
  Saturation Dynamic : simulink/Discontinuities/Saturation Dynamic  OutMin=[]  OutMax=[]  OutDataTypeStr=Inherit: Same as second input  OutDataType=fixdt(1, 16)  OutScaling=2^-10  DoSatur=off
  Switch{,1..4,7} (6 alike) : Switch  Criteria=u2 ~= 0
  Switch Case Action Subsystem : Subsystem  TreatAsAtomicUnit=on
  Switch{5..6,8..15} (10 alike) : Switch  Criteria=u2 > Threshold
  Terminator3 : Terminator
  Timer : hcu_lib/Basic_Blocks/Timer
  Unit Delay : UnitDelay  SampleTime=-1  HasFrameUpgradeWarning=on
  Unit Delay1 : UnitDelay  SampleTime=-1  HasFrameUpgradeWarning=on
  VTQD_CreepEnable_flg : Outport
  VTQD_CreepWhlTqDem_Nm : Outport  Port=2
  VTQD_CreepPrLoadEnable_flg : Outport  Port=3
  VTQD_OPDOn2Off_flg : Outport  Port=4
  VTQD_CreepProtTqEn_flg : Outport  Port=5
  VTQD_VehActSpd_kph : Outport  Port=6
  VTQD_CreepBaseTqD_Nm : Outport  Port=7
  VTQD_CreepBaseTqR_Nm : Outport  Port=8
  VTQD_HighBPSPosn_flg : Outport  Port=9
  wires:
  [VTQD_CreepTotalOfstTq_Nm] -> Add2/2
  If Action Subsystem1/1(VTQD_CreepTotalOfstTq_Nm) -> [VTQD_CreepTotalOfstTq_Nm]  "VTQD_CreepTotalOfstTq_Nm"
  [VTQD_ActBPSPosn_pct] -> If Action Subsystem1/6(VTQD_ActBPSPosn_pct)
  [task_time_s] -> If Action Subsystem1/7(task_time_s)
  [VTQD_CreepDeltaTq_Nm] -> If Action Subsystem1/5(VTQD_CreepDeltaTq_Nm)
  task_time_s/1 -> [task_time_s]
  [VTQD_CreepIterm_c] -> If Action Subsystem1/4(VTQD_CreepIterm_c)
  [VTQD_CreepPterm_c] -> If Action Subsystem1/3(VTQD_CreepPterm_c)
  [VTQD_CreepErrSpd_kph] -> If Action Subsystem1/2(VTQD_CreepErrSpd_kph)
  [VTQD_ActBPSPosnInRange_flg] -> If Action Subsystem1/1(VTQD_ActBPSPosnInRange_flg)
  AND6/1 -> [VTQD_ActBPSPosnInRange_flg]  "VTQD_ActBPSPosnInRange_flg"
  [VTQD_CreepEnable_flg] -> If Action Subsystem1/9(VTQD_CreepEnable_flg)
  NOT4/1 -> Logical Operator3/2
  [VTQD_OPDOn2Off_flg] -> NOT4/1
  NOT3/1 -> Logical Operator3/8
  NOT/1 -> Logical Operator3/7
  Merge/1 -> [VTQD_CreepFinalSpd_kph]  "VTQD_CreepFinalSpd_kph"
  Switch Case Action Subsystem/1(Out1) -> Merge/2
  If Action Subsystem/1(Out1) -> Merge/1
  If/2 -> Switch Case Action Subsystem/Action
  If/1 -> If Action Subsystem/Action
  Equal12/1 -> If/2
  Constant2/1 -> Equal12/2
  [VTQD_GearActualPosn_enum] -> Equal12/1
  Equal13/1 -> If/1
  Constant12/1 -> Equal13/2
  [VTQD_GearActualPosn_enum] -> Equal13/1
  [VTQD_HighBPSPosn_flg] -> OR1/2
  [VVMC_ADASActive_flg] -> NOT3/1
  [VTQD_RBCActive_flg] -> NOT/1
  [VTQD_CreepEnSpd_kph] -> Equal9/2
  VVMC_ADASActive_flg/1 -> [VVMC_ADASActive_flg]
  VINP_FrRBCActive_flg/1 -> [VINP_FrRBCActive_flg]
  VINP_RrRBCActive_flg/1 -> [VINP_RrRBCActive_flg]
  OR1/1 -> [VTQD_CreepDisable_flg]  "VTQD_CreepDisable_flg"
  [VTQD_CreepDisable_flg] -> SR_Latch/2
  [VTQD_RegenMode_enum] -> Equal11/1
  Constant8/1 -> Equal11/2
  [VTQD_CreepON_flg] -> NOT2/1
  Equal10/1 -> OR/2
  Equal6/1 -> OR/1
  Constant7/1 -> Equal10/2
  [VTQD_GearActualPosn_enum] -> Equal10/1
  Constant6/1 -> Equal6/2
  [VTQD_GearActualPosn_enum] -> Equal6/1
  [VTQD_LowIdleAccPedal_flg] -> NOT1/1
  [VTQD_LowIdleAccPedal_flg] -> AND2/2
  GreaterThan1/1 -> AND2/1
  [VTQD_CreepDisSpd_kph] -> GreaterThan1/2
  [VTQD_VehActSpd_kph] -> GreaterThan1/1
  Unit Delay/1 -> GreaterThan/2
  [VTQD_CreepWhlTqDem_Nm] -> Unit Delay/1
  [VTQD_PedalMapWhlTq_Nm] -> GreaterThan/1
  VTQD_PedalMapWhlTq_Nm/1 -> [VTQD_PedalMapWhlTq_Nm]
  [VTQD_LowBPSPosn_flg] -> Logical Operator3/4
  VTQD_ActBPSPosn_pct/1 -> [VTQD_ActBPSPosn_pct]
  Equal7/1 -> Logical Operator5/1
  [VTQD_GearActualPosn_enum] -> Equal8/1
  Equal8/1 -> Logical Operator5/2
  Constant20/1 -> Equal7/2
  Constant21/1 -> Equal8/2
  [VTQD_GearActualPosn_enum] -> Equal7/1
  [VTQD_LowIdleAccPedal_flg] -> Logical Operator3/5
  [VTQD_VehActSpd_kph] -> Equal9/1
  Logical Operator5/1 -> Logical Operator3/3
  Equal9/1 -> Logical Operator3/6
  VTQD_RegenMode_enum/1 -> [VTQD_RegenMode_enum]
  Constant34/1 -> LiuzgSwitch1/3
  Constant33/1 -> LiuzgSwitch1/1
  VTQD_TMRotateDirction_enum/1 -> [VTQD_TMRotateDirction_enum]
  [VTQD_TMRotateDirction_enum] -> Equal1/1
  Constant3/1 -> Equal/2
  Equal/1 -> Logical Operator/1
  [VTQD_GearActualPosn_enum] -> Equal/1
  LiuzgSwitch1/1 -> [VTQD_VehActSpdGain_gain]  "VTQD_VehActSpdGain_gain"
  Equal3/1 -> Logical Operator2/2
  Constant30/1 -> Equal1/2
  Equal1/1 -> Logical Operator/2
  Constant31/1 -> Equal2/2
  Equal2/1 -> Logical Operator2/1
  Logical Operator2/1 -> Logical Operator1/2
  Logical Operator1/1 -> LiuzgSwitch1/2
  Logical Operator/1 -> Logical Operator1/1
  [VTQD_GearActualPosn_enum] -> Equal2/1
  [VTQD_TMRotateDirction_enum] -> Equal3/1
  Constant32/1 -> Equal3/2
  VTQD_LowIdleAccPedal_flg/1 -> [VTQD_LowIdleAccPedal_flg]
  VTQD_CreepON_flg/1 -> [VTQD_CreepON_flg]
  Logical Operator3/1 -> SR_Latch/1
  VTQD_GearActualPosn_enum/1 -> [VTQD_GearActualPosn_enum]
  VINP_VehSpeed_kph/1 -> [VINP_VehSpeed_kph]
  SR_Latch3/1 -> Terminator3/1
  Equal14/1 -> Logical Operator3/9
  Switch/1 -> Switch4/3
  [VTQD_CreepEnable_flg] -> Switch/2
  Constant15/1 -> Switch/3
  [VTQD_LoSpdBrkCtrl_flg] -> NOT9/1
  NOT9/1 -> Logical Operator3/10
  VTQD_LoSpdBrkCtrl_flg/1 -> [VTQD_LoSpdBrkCtrl_flg]
  [VTQD_CreepDisable_flg] -> If Action Subsystem1/8(VTQD_CreepDisable_flg)
  VINP_AVHActive_flg/1 -> [VINP_AVHActive_flg]
  VTQD_APSReq_enum/1 -> [VTQD_APSReq_enum]
  VVMC_APSSpeedCMD_kph/1 -> [VVMC_APSSpeedCMD_kph]
  VVMC_APSActive_flg/1 -> [VVMC_APSActive_flg]
  Switch1/1 -> If Action Subsystem/1(In1)
  [VTQD_CreepTargetSpdD_kph] -> Switch1/3
  [VVMC_APSActive_flg] -> Switch1/2
  [VVMC_APSActive_flg] -> Switch2/2
  Switch2/1 -> Switch Case Action Subsystem/1(In1)
  Constant10/1 -> Switch2/3
  [VVMC_APSActive_flg] -> OR3/1
  [VTQD_CreepON_flg] -> OR3/2
  OR3/1 -> Logical Operator3/1
  NOT2/1 -> AND/2
  AND/1 -> OR1/1
  [VVMC_APSActive_flg] -> NOT5/1
  NOT5/1 -> AND/1
  [VTQD_CreepBaseTqD_Nm] -> Switch3/3
  [VTQD_CreepBaseTqR_Nm] -> Switch3/1
  Switch3/1 -> Add2/1  "VTQD_ActCreepBaseTq_Nm"
  Constant9/1 -> Equal16/2
  [VTQD_GearActualPosn_enum] -> Equal16/1
  Equal16/1 -> Switch3/2
  Timer/1 -> [VTQD_CreepPreloadTime_s], Relational Operator/1  "VTQD_CreepPreloadTime_s"
  [task_time_s] -> Timer/3
  Relational Operator/1 -> [VTQD_CreepEnable_flg], VTQD_CreepEnable_flg/1  "VTQD_CreepEnable_flg"
  SR_Latch/1 -> VTQD_CreepPrLoadEnable_flg/1, [VTQD_CreepPrLoadEnable_flg], NOT8/1, Timer/1  "VTQD_CreepPrLoadEnable_flg"
  NOT8/1 -> Timer/2
  [VTQD_CreepEnable_flg] -> NOT10/1
  NOT10/1 -> AND3/2
  [VTQD_CreepPreloadTq_Nm] -> Switch4/1
  [VTQD_CreepPrLoadEnable_flg] -> AND3/1
  AND3/1 -> Switch4/2
  [VTQD_OPDOn2Off_flg] -> If Action Subsystem1/10(VTQD_OPDOn2Off)
  [VINP_VehSpeed_kph] -> Equal17/1
  Constant23/1 -> Equal17/2
  Equal17/1 -> AND3/3
  AND1/1 -> OR1/3
  AND2/1 -> OR1/4
  OR/1 -> OR1/5
  [VVMC_ADASActive_flg] -> OR1/8
  [VTQD_LoSpdBrkCtrl_flg] -> OR1/10
  VTQD_RDCActive_enum/1 -> [VTQD_RDCActive_enum]
  [VTQD_RDCActive_enum] -> Equal14/1
  Constant17/1 -> Equal14/2
  Constant24/1 -> Equal18/2
  [VTQD_RDCActive_enum] -> Equal18/1
  Equal18/1 -> OR1/9
  [VINP_AVHActive_flg] -> OR1/11
  Equal11/1 -> OR4/1
  [VTQD_GearActualPosn_enum] -> Equal19/1
  Constant25/1 -> Equal19/2
  Equal19/1 -> OR4/2
  VVMC_APSReq_enum/1 -> [VVMC_APSReq_enum]
  Equal22/1 -> Switch6/2
  Constant29/1 -> Switch6/1
  Switch6/1 -> [VTQD_CreepEnSpd_kph]  "VTQD_CreepEnSpd_kph"
  Constant36/1 -> Equal22/2
  Switch5/1 -> [VTQD_CreepDisSpd_kph]  "VTQD_CreepDisSpd_kph"
  Constant35/1 -> Equal21/2
  [VTQD_GearActualPosn_enum] -> Equal22/1
  Add1/1 -> Switch5/1
  [VTQD_GearActualPosn_enum] -> Equal21/1
  Equal21/1 -> Switch5/2
  Constant27/1 -> Add1/1
  Add4/1 -> Switch5/3
  Constant13/1 -> Add4/1
  Constant26/1 -> Add4/2
  Constant28/1 -> Add1/2
  [VVMC_APSSpeedCMD_kph] -> Relational Operator1/1
  [VVMC_APSActive_flg] -> AND5/1
  Constant1/1 -> Relational Operator1/2
  Equal20/1 -> OR5/2
  OR5/1 -> AND5/2
  Constant5/1 -> Equal20/2
  [VVMC_APSReq_enum] -> Equal20/1
  Relational Operator1/1 -> OR5/1
  AND7/1 -> VTQD_CreepProtTqEn_flg/1, [VTQD_CreepProtTqEn_flg]  "VTQD_CreepProtTqEn_flg"
  Equal25/1 -> Logical Operator6/1
  [VTQD_GearActualPosn_enum] -> Equal25/1
  [VTQD_CreepProtTq_Nm] -> Relational Operator2/1
  Constant38/1 -> Equal25/2
  Relational Operator2/1 -> AND7/1
  [VTQD_CreepActWhlTqDem_Nm] -> Relational Operator2/2
  [VTQD_TMRotateDirction_enum] -> Equal26/1
  Constant39/1 -> Equal26/2
  Logical Operator4/1 -> OR6/1
  [VTQD_GearActualPosn_enum] -> Equal23/1
  [VTQD_TMRotateDirction_enum] -> Equal24/1
  Constant11/1 -> Equal23/2
  Equal23/1 -> Logical Operator4/1
  Equal24/1 -> Logical Operator4/2
  Constant37/1 -> Equal24/2
  OR6/1 -> AND7/2
  Equal26/1 -> Logical Operator6/2
  Logical Operator6/1 -> OR6/2
  Switch4/1 -> [VTQD_CreepActWhlTqDem_Nm], Switch7/3  "VTQD_CreepActWhlTqDem_Nm"
  [VTQD_CreepProtTqEn_flg] -> Switch7/2
  Switch7/1 -> VTQD_CreepWhlTqDem_Nm/1, [VTQD_CreepWhlTqDem_Nm]  "VTQD_CreepWhlTqDem_Nm"
  [VTQD_CreepProtTq_Nm] -> Switch7/1
  Relational Operator4/1 -> AND8/2
  NOT7/1 -> AND8/1
  SR_Latch1/1 -> [VTQD_RBCActive_flg]  "VTQD_RBCActive_flg"
  AND8/1 -> SR_Latch1/2  "VTQD_RBCActiveRec_flg"
  Constant41/1 -> Relational Operator4/2
  OR7/1 -> NOT7/1, SR_Latch1/1
  [VINP_FrEDURealTMTq_Nm] -> Relational Operator4/1
  Constant40/1 -> Relational Operator3/2
  [VINP_RrEDURealTMTq_Nm] -> Relational Operator3/1
  Relational Operator3/1 -> AND8/3
  [VINP_RrRBCActive_flg] -> OR7/1
  [VINP_FrRBCActive_flg] -> OR7/2
  VINP_RrEDURealTMTq_Nm/1 -> [VINP_RrEDURealTMTq_Nm]
  " VINP_FrEDURealTMTq_Nm"/1 -> [VINP_FrEDURealTMTq_Nm]
  [VVMC_EstSlope_Deg] -> Relay/1
  Relay/1 -> Data Type Conversion/1
  Ground2/1 -> [VTQD_OPDOn2Off_flg], VTQD_OPDOn2Off_flg/1  "VTQD_OPDOn2Off_flg"
  VTQD_PreLoadPreEn_flg/1 -> [VTQD_PreLoadPreEn_flg]
  VVMC_EstSlope_Deg/1 -> [VVMC_EstSlope_Deg]
  VPMM_PwrSta_enum/1 -> [VPMM_PwrSta_enum]
  [VPMM_PwrSta_enum] -> Equal30/1
  Equal29/1 -> OR2/2
  [VTQD_GearActualPosn_enum] -> Equal29/1
  Equal4/1 -> GreaterThan3/2, Unit Delay1/1
  Constant4/1 -> Equal4/2
  [VTQD_LowIdleAccPedal_flg] -> NOT6/1
  GreaterThan3/1 -> AND4/2
  Equal30/1 -> AND4/1
  Constant45/1 -> Equal30/2
  Constant44/1 -> Equal29/2
  NOT6/1 -> OR2/1
  [VTQD_RegenMode_enum] -> Equal4/1
  OR2/1 -> SR_Latch3/2
  Unit Delay1/1 -> GreaterThan3/1
  AND4/1 -> SR_Latch3/1
  Constant43/1 -> Equal28/2
  [VVMC_EstSlope_Deg] -> MTQD_CreepBPSDisPosnR_Y_pct/1
  Equal27/1 -> Switch8/2
  MTQD_CreepBPSDisPosn_Y_pct/1 -> Switch9/3  "VTQD_CreepBPSDisPosn_pct"
  [VTQD_ActBPSPosn_pct] -> GreaterThan2/1
  GreaterThan2/1 -> VTQD_HighBPSPosn_flg/1, [VTQD_HighBPSPosn_flg]  "VTQD_HighBPSPosn_flg"
  Switch9/1 -> GreaterThan2/2
  Equal5/1 -> [VTQD_LowBPSPosn_flg]  "VTQD_LowBPSPosn_flg"
  Equal28/1 -> Switch9/2
  [VVMC_EstSlope_Deg] -> MTQD_CreepBPSDisPosn_Y_pct/1
  [VTQD_GearActualPosn_enum] -> Equal28/1
  Constant42/1 -> Equal27/2
  Switch8/1 -> Equal5/2
  [VVMC_EstSlope_Deg] -> MTQD_CreepBPSEnPosnR_Y_pct/1
  MTQD_CreepBPSEnPosn_Y_pct/1 -> Switch8/3  "VTQD_CreepBPSEnPosn_pct"
  MTQD_CreepBPSDisPosnR_Y_pct/1 -> Switch9/1  "VTQD_CreepBPSDisPosnR_pct"
  [VTQD_GearActualPosn_enum] -> Equal27/1
  MTQD_CreepBPSEnPosnR_Y_pct/1 -> Switch8/1  "VTQD_CreepBPSEnPosnR_pct"
  [VTQD_ActBPSPosn_pct] -> Equal5/1
  [VVMC_EstSlope_Deg] -> MTQD_CreepBPSEnPosn_Y_pct/1
  NOT11/1 -> Logical Operator3/11
  [VTQD_PreLoadPreEn_flg] -> NOT11/1
  [VTQD_VehActSpd_kph] -> MTQD_CreepPreloadTime_Y_s/1
  Delay/1 -> Switch10/1
  [VTQD_CreepEnable_flg] -> Delay1/1
  Delay1/1 -> Switch10/2
  MTQD_CreepPreloadTime_Y_s/1 -> Switch10/3  "VTQD_CreepPreloadSetTime_s"
  Switch10/1 -> Delay/1, Relational Operator/2, Timer/4
  MTQD_CreepPterm_Z_Nm/1 -> [VTQD_CreepPterm_c]  "VTQD_CreepPterm_c"
  Add/1 -> [VTQD_CreepErrSpd_kph]  "VTQD_CreepErrSpd_kph"
  [VINP_VehSpeed_kph] -> MTQD_CreepPrelaodTq_Z_Nm/2
  [VVMC_EstSlope_Deg] -> MTQD_CreepBaseTqR_Z_Nm/1
  MTQD_CreepBaseTqD_Z_Nm/1 -> VTQD_CreepBaseTqD_Nm/1, [VTQD_CreepBaseTqD_Nm]  "VTQD_CreepBaseTqD_Nm"
  [VTQD_VehActSpd_kph] -> MTQD_CreepBaseTqD_Z_Nm/2
  MTQD_CreepDeltaTq_Y_Nm/1 -> [VTQD_CreepDeltaTq_Nm]  "VTQD_CreepDeltaTq_Nm"
  [VTQD_VehActSpd_kph] -> Add/2
  [VTQD_VehActSpd_kph] -> MTQD_CreepBaseTqR_Z_Nm/2
  [VTQD_CreepPreloadTime_s] -> MTQD_CreepPrelaodTq_Z_Nm/1
  MTQD_CreepBaseTqR_Z_Nm/1 -> VTQD_CreepBaseTqR_Nm/1, [VTQD_CreepBaseTqR_Nm]  "VTQD_CreepBaseTqR_Nm"
  [VTQD_CreepFinalSpd_kph] -> Add/1
  [VVMC_EstSlope_Deg] -> MTQD_CreepBaseTqD_Z_Nm/1
  MTQD_CreepPrelaodTq_Z_Nm/1 -> [VTQD_CreepPreloadTq_Nm]  "VTQD_CreepPreloadTq_Nm"
  MTQD_CreepProtTq_Y_Nm/1 -> [VTQD_CreepProtTq_Nm]  "VTQD_CreepProtTq_Nm"
  [VTQD_CreepErrSpd_kph] -> MTQD_CreepDeltaTq_Y_Nm/1
  [VVMC_EstSlope_Deg] -> MTQD_CreepProtTq_Y_Nm/1
  [VTQD_GearActualPosn_enum] -> Detect Change/1
  Constant46/1 -> Switch13/3
  [VTQD_OPDHoldEnSpd_kph] -> Switch13/1
  [VTQD_RegenMode_enum] -> Equal33/1
  Constant54/1 -> Equal33/2
  Equal33/1 -> AND16/1
  Switch13/1 -> Switch6/3
  [VVMC_EstSlope_Deg] -> MTQD_OPDHoldEnSpd_Y_kph/1
  MTQD_OPDHoldEnSpd_Y_kph/1 -> [VTQD_OPDHoldEnSpd_kph]  "VTQD_OPDHoldEnSpd_kph"
  [VTQD_LowBPSPosn_flg] -> NOT12/1
  [VTQD_HighBPSPosn_flg] -> NOT13/1
  NOT12/1 -> AND6/1
  NOT13/1 -> AND6/2
  OR4/1 -> OR1/6
  [VTQD_RBCActive_flg] -> OR1/7
  Constant53/1 -> Equal32/2
  [VTQD_APSReqTimer_s] -> Equal32/1
  Equal32/1 -> OR8/2
  Data Type Conversion/1 -> OR8/1  "VTQD_OPDCreepGrade_flg"
  OR8/1 -> OR4/3
  [VTQD_APSReq_enum] -> Equal15/1
  Constant18/1 -> Equal15/2
  Equal15/1 -> AND11/1
  Constant51/1 -> AND11/2
  AND11/1 -> OR1/12
  Equal34/1 -> Logical Operator7/1
  Constant55/1 -> Equal34/2
  [VINP_EPBSta_enum] -> Equal34/1
  Constant16/1 -> Product1/3
  Constant19/1 -> Product1/4
  [VTQD_VehActSpdGain_gain] -> Product/1
  Constant48/1 -> AND10/1
  Constant47/1 -> FirstOrderFilter/3
  Switch11/1 -> VTQD_VehActSpd_kph/1, [VTQD_VehActSpd_kph]  "VTQD_VehActSpd_kph"
  FirstOrderFilter/1 -> [VTQD_RPM2VehSpd_kph]  "VTQD_RPM2VehSpd_kph"
  Product1/1 -> FirstOrderFilter/1
  AND9/1 -> Switch11/2
  [VTQD_RPM2VehSpd_kph] -> Switch11/1
  Product/1 -> Switch11/3
  [VINP_VehSpeed_kph] -> Product/2
  Constant14/1 -> Product1/2
  [VVMC_APSActive_flg] -> AND10/2
  Relay1/1 -> AND9/2
  [task_time_s] -> FirstOrderFilter/2
  AND10/1 -> AND9/1
  [VINP_VehSpeed_kph] -> Relay1/1
  [VTQD_TqTargetShaftSpd_rpm] -> Product1/1
  Constant49/1 -> Switch12/3
  Equal31/1 -> AND12/1
  AND12/1 -> Switch12/2
  Switch12/1 -> [VTQD_CreepTargetSpdD_kph]  "VTQD_CreepTargetSpdD_kph"
  Constant56/1 -> NOT14/1
  NOT14/1 -> AND12/2
  [VTQD_RegenMode_enum] -> Equal31/1
  Constant52/1 -> Equal31/2
  Constant50/1 -> Switch12/1
  Add2/1 -> Saturation Dynamic/2
  Constant22/1 -> Saturation Dynamic/3
  Constant60/1 -> Switch14/1
  Constant59/1 -> Equal36/2
  Switch14/1 -> Saturation Dynamic/1  "VTQD_CreepUpLimitTq_Nm"
  [VTQD_GearActualPosn_enum] -> Equal35/1
  Constant58/1 -> Equal35/2
  AND13/1 -> Switch14/2
  Equal35/1 -> AND13/1
  Equal36/1 -> AND13/2
  Constant57/1 -> Switch14/3
  Saturation Dynamic/1 -> Switch/1
  VINP_EPBSta_enum/1 -> [VINP_EPBSta_enum]
  VTQD_TqTargetShaftSpd_rpm/1 -> [VTQD_TqTargetShaftSpd_rpm]
  VTQD_APSReqTimer_s/1 -> [VTQD_APSReqTimer_s]
  [VTQD_VehActSpd_kph] -> GreaterThan4/1
  Constant61/1 -> GreaterThan4/2
  NOT1/1 -> AND1/2
  Switch15/1 -> AND1/1
  VTQD_OPDHoldEnRel_flg/1 -> [VTQD_OPDHoldEnRel_flg]
  [VTQD_OPDHoldEnRel_flg] -> Switch15/1
  [VTQD_GearActualPosn_enum] -> Equal37/1
  Constant62/1 -> Equal37/2
  AND14/1 -> Switch15/2
  GreaterThan4/1 -> AND14/2
  Equal37/1 -> AND14/1
  [VVMC_APSSpeedCMD_kph] -> Switch1/1
  [VVMC_APSSpeedCMD_kph] -> Switch2/1
  GreaterThan/1 -> AND15/2
  AND15/1 -> Switch15/3
  NOT15/1 -> AND15/1
  [VVMC_APSActive_flg] -> NOT15/1
  [VTQD_ActAPSPosn_pct] -> Relational Operator5/1
  Constant63/1 -> Relational Operator5/2
  Relational Operator5/1 -> AND14/3
  VTQD_ActAPSPosn_pct/1 -> [VTQD_ActAPSPosn_pct]
  VVMC_CAASActive_flg/1 -> [VVMC_CAASActive_flg]
  AND5/1 -> OR1/16
  [VVMC_CAASActive_flg] -> OR1/15
  [VTQD_RegenMode_enum] -> Equal38/1
  Constant64/1 -> Equal38/2
  Detect Change/1 -> OR9/2
  OR9/1 -> OR1/13
  Equal38/1 -> Detect Increase/1
  Detect Increase/1 -> OR9/1
  [VTQD_VehActSpd_kph] -> MTQD_CreepIterm_Z_Nm/1
  MTQD_CreepIterm_Z_Nm/1 -> [VTQD_CreepIterm_c]  "VTQD_CreepIterm_c"
  [VTQD_CreepErrSpd_kph] -> MTQD_CreepIterm_Z_Nm/2
  [VVMC_APSReq_enum] -> Equal39/1
  Constant65/1 -> Equal39/2
  Equal39/1 -> OR5/3
  [VTQD_RegenMode_enum] -> Equal36/1
  [VTQD_VehActSpd_kph] -> MTQD_CreepPterm_Z_Nm/1
  [VTQD_CreepErrSpd_kph] -> MTQD_CreepPterm_Z_Nm/2
  [VDDM_EPB1CSErrCFS_flg] -> Logical Operator10/1
  Logical Operator8/1 -> Logical Operator7/2
  Logical Operator7/1 -> OR1/14
  [VDDM_EPBSigErrCFS_flg] -> Logical Operator11/1
  Logical Operator10/1 -> Logical Operator7/4
  Logical Operator11/1 -> Logical Operator7/5
  [VDDM_EPB1NoComCFS_flg] -> Logical Operator8/1
  Logical Operator9/1 -> Logical Operator7/3
  [VDDM_EPB1RCErrCFS_flg] -> Logical Operator9/1
  NOT16/1 -> OR4/4
  [VVMC_APSActive_flg] -> NOT16/1
  VDDM_EPB1RCErrCFS_flg/1 -> [VDDM_EPB1RCErrCFS_flg]
  VDDM_EPBSigErrCFS_flg/1 -> [VDDM_EPBSigErrCFS_flg]
  VDDM_EPB1NoComCFS_flg/1 -> [VDDM_EPB1NoComCFS_flg]
  VDDM_EPB1CSErrCFS_flg/1 -> [VDDM_EPB1CSErrCFS_flg]
  [VVMC_APSActive_flg] -> NOT18/1
  NOT18/1 -> AND13/3
  AND16/1 -> Switch13/2
  [VVMC_APSActive_flg] -> NOT17/1
  NOT17/1 -> AND16/2
